simulink model "intgratedMCUSlugs"  (Simulink 7.8)
settings: Solver=FixedStepDiscrete  SolverMode=SingleTasking  StartTime=0.0  StopTime=10.0  FixedStep=0.001  RelTol=1e-3
InitFcn:
  | mcuInit
undefined symbols (not defined in the file): accBiasRateLimit, apSampleTime, barAdjust, baroCutoff, baroCutTemp, baroOffset, baroScale, barTGain1, barTGain2, barTMean1, barTMean2, baseHeight, baseTemp, bda, bde, bdr, bdt, bICda, bICde, bICdr, bICdt, bpan, bPWMpan, bPWMtilt, broll, btilt, changeZoom, controlMCUInit, cubeAccelGain16405, cubeGyroGain16405, cubeMagGain16405, daTrimMax, daTrimMin, deTrimMax, deTrimMin, DiscIntNeverNeededParam, drTrimMax, drTrimMin, dtTrimMax, dtTrimMin, Function_Update, gaind, getCubeData, getGpsMainData, getGPSRawData, getGpsUbloxMainData, getGSLocation, getISRLocation, getMidLevelCommands, getMobileLocation, getPassValues, getRangeOfParams, getRTB, gpsParse, gsRead, gyroBiasRateLimit, hil_getEuler, hil_getRates, hil_getRawRead, hil_getVned ... (+89)
libraries: dsPICdrivers x105, simulink x14, SLUGS_Library x12, aerolibconvert2 x5, aerolibutil x4, aerolibtransform2 x3, dspmtrx3 x3, aerolibobsolete x3
(part 1 of 6)
settings Model: Creator=Marcello G  LastModifiedBy=Marcello G
settings OptimizationCC: OptimizeModelRefInitCode=on  LifeSpan=1
settings DebuggingCC: ParameterPrecisionLossMsg=none
settings HardwareCC: ProdBitPerInt=16  ProdBitPerPointer=16  ProdEndianess=LittleEndian  ProdWordSize=16  ProdHWDeviceType=16-bit Generic
settings RTWCC: SystemTargetFile=dspic.tlc  MakeCommand=make_CreateMPLAB  TemplateMakefile=dspic_pic30_gcc.tmf  PostCodeGenCommand=dsPIC_Compile()  Description=Embedded Target for Microchip dsPIC (real-time)  ProcessScript=dspic_make_rtw_hook
settings CodeAppCC: IgnoreCustomStorageClasses=off
settings STFCustomTargetCC: IncludeMdlTerminateFcn=off  GeneratePreprocessorConditionals=Use local settings  CombineOutputUpdateFcns=on  SuppressErrorStatus=on  ERTCustomFileBanners=on  SupportContinuousTime=off  SupportNonInlinedSFcns=off  SystemTargetFile=dspic.tlc
settings ERTTargetCC: MultiwordLength=2048  ParMdlRefBuildCompliant=off  CompOptLevelCompliant=off  ConcurrentExecutionCompliant=off  IncludeMdlTerminateFcn=off  SuppressErrorStatus=on  ERTFirstTimeCompliant=off  ModelStepFunctionPrototypeControlCompliant=off  CPPClassGenCompliant=off  ExtModeMexFile=ext_serial_win32_comm  InlinedParameterPlacement=NonHierarchical  ERTSrcFileBannerTemplate=dsPIC_code_template.cgt  ERTHdrFileBannerTemplate=dsPIC_code_template.cgt  ERTDataSrcFileTemplate=dsPIC_code_template.cgt  ERTDataHdrFileTemplate=dsPIC_code_template.cgt  ERTCustomFileTemplate=dsPIC_main.tlc  ConvertIfToSwitch=off  SuppressUnreachableDefaultCases=off
settings CustomProperty: DataType=string  Value=D:\MATLAB~1\bin\win64\gmake

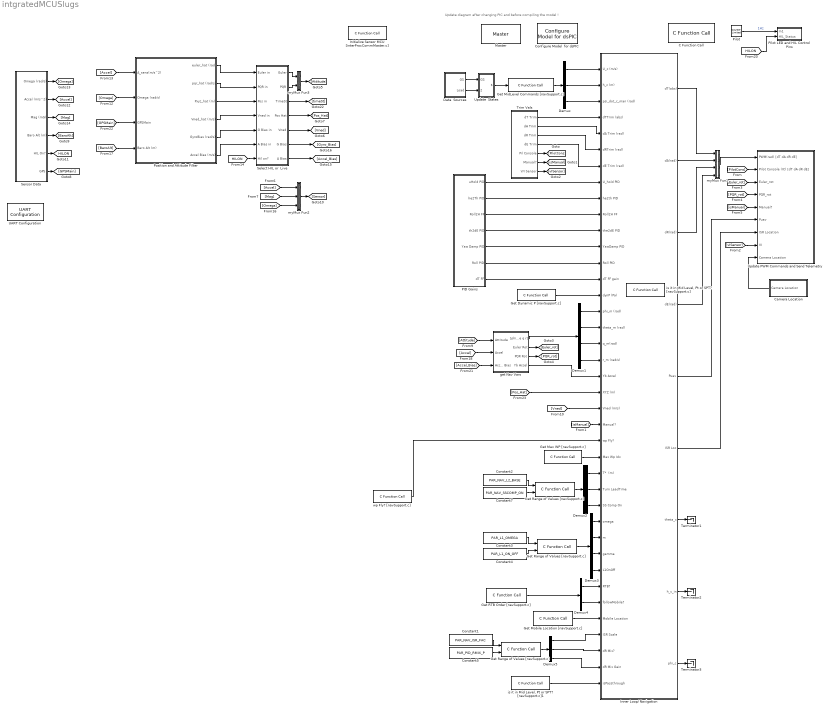
== system intgratedMCUSlugs ==
  note: Update diagram after changing PIC and before compiling the model !
  C Function Call : dsPICdrivers/OTHERS/C Function Call  Tag=dsPIC_dsPIC_CFunctionCall  FctUpdate=None  fctName='Function_Update'  INPUT_SIZE=1  INPUT1=--  INPUT2=--  INPUT3=--  OUTPUT_SIZE=1  OUTPUT1=--  SampleTime=-1  InputType=[]  OutputType=[]  FctDeclaration=extern void Function_Update();  FctCall=Function_Update();  OrderingInOutPopup=None  FctStart=Start Function (Call once and only once)  FctStart_Name='controlMCUInit'  FctStart_Declaration=inline extern void controlMCUInit();  FctStart_Call=controlMCUInit();  FctInit=None  FctInit_Name=Init_Reset  FctInit_Declaration=inline extern void Init_Reset();  FctInit_Call=Init_Reset();  PinDigitalInput=[]  PinDigitalOutput=[]  AnalogueInput=[]
  Camera Location : Subsystem
  Configure Model  for dsPIC : dsPICdrivers/Simulink Configuration/Configure Model  for dsPIC
  Constant1 : Constant  Value=PAR_NAV_ISR_FAC  OutDataTypeStr=uint8
  Constant2 : Constant  Value=PAR_NAV_L2_BASE  OutDataTypeStr=uint8
  Constant3 : Constant  Value=PAR_L1_OMEGA  OutDataTypeStr=uint8
  Constant4 : Constant  Value=PAR_L1_ON_OFF  OutDataTypeStr=uint8
  Constant5 : Constant  Value=PAR_PID_RMIX_P  OutDataTypeStr=uint8
  Constant7 : Constant  Value=PAR_NAV_SSCOMP_ON  OutDataTypeStr=uint8
  Data  Sources : Subsystem
  Demux : Demux  Outputs=3
  Demux1 : Demux
  Demux2 : Demux  Outputs=3
  Demux3 : Demux
  Demux4 : Demux  Outputs=2
  Demux5 : Demux  Outputs=3
  Get Dynamic P [navSupport.c] : dsPICdrivers/OTHERS/C Function Call  Tag=dsPIC_dsPIC_CFunctionCall  FctUpdate=Output Function  fctName='getDynamic'  INPUT_SIZE=1  INPUT1=--  INPUT2=--  INPUT3=--  OUTPUT_SIZE=1  OUTPUT1=real32  SampleTime=.01  InputType=[ ]  OutputType=[ 7 ]  FctDeclaration=extern real32_T getDynamic();  FctCall=%y1 = getDynamic();  OrderingInOutPopup=None  FctStart=None  FctStart_Name=Init_onlyOnce  FctStart_Declaration=inline extern void Init_onlyOnce();  FctStart_Call=Init_onlyOnce();  FctInit=None  FctInit_Name=Init_Reset  FctInit_Declaration=inline extern void Init_Reset();  FctInit_Call=Init_Reset();  PinDigitalInput=[]  PinDigitalOutput=[]  AnalogueInput=[]
  Get Max WP [navSupport.c] : dsPICdrivers/OTHERS/C Function Call  Tag=dsPIC_dsPIC_CFunctionCall  FctUpdate=Output Function  fctName='getMaxWp'  INPUT_SIZE=1  INPUT1=--  INPUT2=--  INPUT3=--  OUTPUT_SIZE=1  OUTPUT1=uint8  SampleTime=.01  InputType=[ ]  OutputType=[ 2 ]  FctDeclaration=extern uint8_T getMaxWp();  FctCall=%y1 = getMaxWp();  OrderingInOutPopup=None  FctStart=None  FctStart_Name=Init_onlyOnce  FctStart_Declaration=inline extern void Init_onlyOnce();  FctStart_Call=Init_onlyOnce();  FctInit=None  FctInit_Name=Init_Reset  FctInit_Declaration=inline extern void Init_Reset();  FctInit_Call=Init_Reset();  PinDigitalInput=[]  PinDigitalOutput=[]  AnalogueInput=[]
  Get MidLevel Commands [navSupport.c] : dsPICdrivers/OTHERS/C Function Call  Tag=dsPIC_dsPIC_CFunctionCall  FctUpdate=Output Function  fctName='getMidLevelCommands'  INPUT_SIZE=1  INPUT1=--  INPUT2=--  INPUT3=--  OUTPUT_SIZE=3  OUTPUT1=real32  SampleTime=.01  InputType=[ ]  OutputType=[ 7 ]  FctDeclaration=extern void getMidLevelCommands(real32_T* y1);  FctCall=getMidLevelCommands(*%y1);  OrderingInOutPopup=Input  FctStart=None  FctStart_Name=Init_onlyOnce  FctStart_Declaration=inline extern void Init_onlyOnce();  FctStart_Call=Init_onlyOnce();  FctInit=None  FctInit_Name=Init_Reset  FctInit_Declaration=inline extern void Init_Reset();  FctInit_Call=Init_Reset();  PinDigitalInput=[]  PinDigitalOutput=[]  AnalogueInput=[]
  "Get Mobile Location [navSupport.c] " : dsPICdrivers/OTHERS/C Function Call  Tag=dsPIC_dsPIC_CFunctionCall  FctUpdate=Output Function  fctName='getMobileLocation'  INPUT_SIZE=1  INPUT1=--  INPUT2=--  INPUT3=--  OUTPUT_SIZE=2  OUTPUT1=real32  SampleTime=.01  InputType=[ ]  OutputType=[ 7 ]  FctDeclaration=extern void getMobileLocation(real32_T* y1);  FctCall=getMobileLocation(*%y1);  OrderingInOutPopup=None  FctStart=None  FctStart_Name=Init_onlyOnce  FctStart_Declaration=inline extern void Init_onlyOnce();  FctStart_Call=Init_onlyOnce();  FctInit=None  FctInit_Name=Init_Reset  FctInit_Declaration=inline extern void Init_Reset();  FctInit_Call=Init_Reset();  PinDigitalInput=[]  PinDigitalOutput=[]  AnalogueInput=[]
  Get RTB Order [navSupport.c] : dsPICdrivers/OTHERS/C Function Call  Tag=dsPIC_dsPIC_CFunctionCall  FctUpdate=Output Function  fctName='getRTB'  INPUT_SIZE=1  INPUT1=--  INPUT2=--  INPUT3=--  OUTPUT_SIZE=2  OUTPUT1=uint8  SampleTime=.01  InputType=[ ]  OutputType=[ 2 ]  FctDeclaration=extern void getRTB(uint8_T* y1);  FctCall=getRTB(*%y1);  OrderingInOutPopup=None  FctStart=None  FctStart_Name=Init_onlyOnce  FctStart_Declaration=inline extern void Init_onlyOnce();  FctStart_Call=Init_onlyOnce();  FctInit=None  FctInit_Name=Init_Reset  FctInit_Declaration=inline extern void Init_Reset();  FctInit_Call=Init_Reset();  PinDigitalInput=[]  PinDigitalOutput=[]  AnalogueInput=[]
  Get Range of Values [navSupport.c] : dsPICdrivers/OTHERS/C Function Call  Tag=dsPIC_dsPIC_CFunctionCall  FctUpdate=Output Function  fctName='getRangeOfParams'  INPUT_SIZE=1  INPUT1=uint8  INPUT2=uint8  INPUT3=--  OUTPUT_SIZE=3  OUTPUT1=real32  SampleTime=.01  InputType=[ 2 2 ]  OutputType=[ 7 ]  FctDeclaration=extern void getRangeOfParams(uint8_T u1, uint8_T u2,real32_T* y1);  FctCall=getRangeOfParams(%u1, %u2, *%y1);  OrderingInOutPopup=None  FctStart=None  FctStart_Name=Init_onlyOnce  FctStart_Declaration=inline extern void Init_onlyOnce();  FctStart_Call=Init_onlyOnce();  FctInit=None  FctInit_Name=Init_Reset  FctInit_Declaration=inline extern void Init_Reset();  FctInit_Call=Init_Reset();  PinDigitalInput=[]  PinDigitalOutput=[]  AnalogueInput=[]
  "Get Range of Values [navSupport.c] " : dsPICdrivers/OTHERS/C Function Call  Tag=dsPIC_dsPIC_CFunctionCall  FctUpdate=Output Function  fctName='getRangeOfParams'  INPUT_SIZE=1  INPUT1=uint8  INPUT2=uint8  INPUT3=--  OUTPUT_SIZE=4  OUTPUT1=real32  SampleTime=.01  InputType=[ 2 2 ]  OutputType=[ 7 ]  FctDeclaration=extern void getRangeOfParams(uint8_T u1, uint8_T u2,real32_T* y1);  FctCall=getRangeOfParams(%u1, %u2, *%y1);  OrderingInOutPopup=None  FctStart=None  FctStart_Name=Init_onlyOnce  FctStart_Declaration=inline extern void Init_onlyOnce();  FctStart_Call=Init_onlyOnce();  FctInit=None  FctInit_Name=Init_Reset  FctInit_Declaration=inline extern void Init_Reset();  FctInit_Call=Init_Reset();  PinDigitalInput=[]  PinDigitalOutput=[]  AnalogueInput=[]
  "Get Range of Values [navSupport.c]   " : dsPICdrivers/OTHERS/C Function Call  Tag=dsPIC_dsPIC_CFunctionCall  FctUpdate=Output Function  fctName='getRangeOfParams'  INPUT_SIZE=1  INPUT1=uint8  INPUT2=uint8  INPUT3=--  OUTPUT_SIZE=3  OUTPUT1=real32  SampleTime=.01  InputType=[ 2 2 ]  OutputType=[ 7 ]  FctDeclaration=extern void getRangeOfParams(uint8_T u1, uint8_T u2,real32_T* y1);  FctCall=getRangeOfParams(%u1, %u2, *%y1);  OrderingInOutPopup=None  FctStart=None  FctStart_Name=Init_onlyOnce  FctStart_Declaration=inline extern void Init_onlyOnce();  FctStart_Call=Init_onlyOnce();  FctInit=None  FctInit_Name=Init_Reset  FctInit_Declaration=inline extern void Init_Reset();  FctInit_Call=Init_Reset();  PinDigitalInput=[]  PinDigitalOutput=[]  AnalogueInput=[]
  Initialize Sensor MCU [interProcCommMaster.c] : dsPICdrivers/OTHERS/C Function Call  Tag=dsPIC_dsPIC_CFunctionCall  FctUpdate=None  fctName='Function_Update'  INPUT_SIZE=1  INPUT1=--  INPUT2=--  INPUT3=--  OUTPUT_SIZE=1  OUTPUT1=--  SampleTime=inf  InputType=[]  OutputType=[]  FctDeclaration=extern void Function_Update();  FctCall=Function_Update();  OrderingInOutPopup=None  FctStart=Start Function (Call once and only once)  FctStart_Name='sensorMCUInit'  FctStart_Declaration=inline extern void sensorMCUInit();  FctStart_Call=sensorMCUInit();  FctInit=None  FctInit_Name=Init_Reset  FctInit_Declaration=inline extern void Init_Reset();  FctInit_Call=Init_Reset();  PinDigitalInput=[]  PinDigitalOutput=[]  AnalogueInput=[]
  Inner Loop/ Navigation : Subsystem
  Master : dsPICdrivers/Master  Tag=dsPIC_MASTER  Priority=1  TimeStepType=Timer1  picType=33fJ256MC710  fcy=40000000  Quartz_33f=12e6  PLLActive_33f=on  fcyDesired_33f=40000000  tmr1="[1  39999  0]"  tmr1Info="Time Step : 0.001  ;   Error : 0%  PR1=39999"  tmr2345="[8  0  0  0  0  0  0  0]"  tmr2345cfg=[-1 -1 -1 -1 -1 -1 -1 -1]  IOautoConf=on  typePort="[ 0   0   0   0   0   0   0   0   0   0   0   0   0   0   9   0   0   0   0   0   0   0  10   0   8   8   8   8   0   0   0   0   0   0   0   0   0   0   0   0   0   0   0   0   0   0   0   0   0   0   9   0   0   0   0   0   6   6   6   6   6   0   6   6  11   0  11   0  11   0  11   0   0  10   0   0   0   0   0   0   0   0   4   0   0   0   0   0   0   0   0   0   0   0   0   0   0   0   0   0   0   0   0  10  10  10   0   0   0   0   0  10 ]"  TRIS="[ 65535  65471  65535  65535  65023  65535  31871 ]"  ADPCFG=2097216  MasterBusyPort=None  MasterOverloadPort=None  FOSC=External Clock  ClockSwitchMonitor=Both disabled  TempProtection_33f=TEMP_ON  FPBOR=<empty>  PWRT=disable  MCLR=<empty>  ICD=ICS_PGD2  JTAGEN=JTAGEN_OFF  PowerSave=off  OverrideFcy=off  NewFcy=1e6  PR2345="[65535  65535  65535  65535  65535  65535  65535  65535]"
  PID Gains : Subsystem
  Pilot : simulink/Sources/Counter Limited  uplimit=1  tsamp=1.0
  Pilot LED and HIL Control Pins : Subsystem
  Position and Attitude Filter : Subsystem
  Select HIL or  Live : Subsystem
  Sensor Data : Subsystem
  Terminator1 : Terminator
  Terminator2 : Terminator
  Terminator3 : Terminator
  Trim Vals : Subsystem
  UART Configuration : dsPICdrivers/Serial PORT/UART Configuration  Tag=dsPIC_config_UART  Priority=2  UART=1  proposed_BAUD=38400  BAUD=38400  ALT_TX_RX=on  InterruptTxWhen=When Transmit Buffer is empty  TXInterruptPri=1  TxBufferSize=32  TXEN=off  InterruptRxWhen=When a character is received  RXInterruptPri=2  RxBufferSize=32  DoNotImplementRxInterrupt=on  DoNotImplementTxInterrupt=on  UxBRG=64  Info="UxBRG = 64   ||  Real Baud : 38462   ||  % error : 0.16026  ||  max 3.8462 Bytes / Step"  RealBaud=0  ERROR=0.16026  BYTES_STEP=3.8462
  Update  States : Subsystem
  Update PWM Commands and Send Telemetry : Subsystem
  get Nav Vars : Subsystem
  "is it in Mid Level, Pt or SPT? [navSupport.c]" : dsPICdrivers/OTHERS/C Function Call  Tag=dsPIC_dsPIC_CFunctionCall  FctUpdate=Output Function  fctName='isPassthrough'  INPUT_SIZE=1  INPUT1=--  INPUT2=--  INPUT3=--  OUTPUT_SIZE=1  OUTPUT1=uint8  SampleTime=0.01  InputType=[ ]  OutputType=[ 2 ]  FctDeclaration=extern uint8_T isPassthrough();  FctCall=%y1 = isPassthrough();  OrderingInOutPopup=None  FctStart=None  FctStart_Name=Init_onlyOnce  FctStart_Declaration=inline extern void Init_onlyOnce();  FctStart_Call=Init_onlyOnce();  FctInit=None  FctInit_Name=Init_Reset  FctInit_Declaration=inline extern void Init_Reset();  FctInit_Call=Init_Reset();  PinDigitalInput=[]  PinDigitalOutput=[]  AnalogueInput=[]
  "is it in Mid Level, Pt or SPT? [navSupport.c]1" : dsPICdrivers/OTHERS/C Function Call  Tag=dsPIC_dsPIC_CFunctionCall  FctUpdate=Output Function  fctName='isPassthrough'  INPUT_SIZE=1  INPUT1=--  INPUT2=--  INPUT3=--  OUTPUT_SIZE=1  OUTPUT1=uint8  SampleTime=0.01  InputType=[ ]  OutputType=[ 2 ]  FctDeclaration=extern uint8_T isPassthrough();  FctCall=%y1 = isPassthrough();  OrderingInOutPopup=None  FctStart=None  FctStart_Name=Init_onlyOnce  FctStart_Declaration=inline extern void Init_onlyOnce();  FctStart_Call=Init_onlyOnce();  FctInit=None  FctInit_Name=Init_Reset  FctInit_Declaration=inline extern void Init_Reset();  FctInit_Call=Init_Reset();  PinDigitalInput=[]  PinDigitalOutput=[]  AnalogueInput=[]
  myMux Fun1 : MATLAB Function  TreatAsAtomicUnit=on
  myMux Fun2 : MATLAB Function  TreatAsAtomicUnit=on
  myMux Fun3 : MATLAB Function  TreatAsAtomicUnit=on
  wp Fly? [navSupport.c] : dsPICdrivers/OTHERS/C Function Call  Tag=dsPIC_dsPIC_CFunctionCall  FctUpdate=Output Function  fctName='isWpFly'  INPUT_SIZE=1  INPUT1=--  INPUT2=--  INPUT3=--  OUTPUT_SIZE=1  OUTPUT1=uint8  SampleTime=.01  InputType=[ ]  OutputType=[ 2 ]  FctDeclaration=extern uint8_T isWpFly();  FctCall=%y1 = isWpFly();  OrderingInOutPopup=None  FctStart=None  FctStart_Name=Init_onlyOnce  FctStart_Declaration=inline extern void Init_onlyOnce();  FctStart_Call=Init_onlyOnce();  FctInit=None  FctInit_Name=Init_Reset  FctInit_Declaration=inline extern void Init_Reset();  FctInit_Call=Init_Reset();  PinDigitalInput=[]  PinDigitalOutput=[]  AnalogueInput=[]
  tag scope: HILON=global
  wires:
  Pilot/1 -> Pilot LED and HIL Control Pins/1(In1)  "1Hz"
  Data  Sources/1(GS) -> Update  States/1(GS)
  Data  Sources/2(Load) -> Update  States/2(Load)
  Demux/1 -> Inner Loop/ Navigation/1(U_c (m/s))
  Demux/2 -> Inner Loop/ Navigation/2(h_c (m))
  Demux/3 -> Inner Loop/ Navigation/3(psi_dot_c_man (rad))
  Get MidLevel Commands [navSupport.c]/1 -> Demux/1
  Trim Vals/4(dE Trim) -> Inner Loop/ Navigation/7(dE Trim (rad))
  Trim Vals/1(dT Trim) -> Inner Loop/ Navigation/4(dTTrim (abs))
  Trim Vals/2(dA Trim) -> Inner Loop/ Navigation/5(dA Trim (rad))
  Trim Vals/3(dR Trim) -> Inner Loop/ Navigation/6(dRTrim (rad))
  PID Gains/1(uHold PID) -> Inner Loop/ Navigation/8(U_hold PID)
  PID Gains/2(he2Th PID) -> Inner Loop/ Navigation/9(he2th PID)
  PID Gains/4(th2dE PID) -> Inner Loop/ Navigation/11(the2dE PID)
  PID Gains/5(Yaw Damp PID) -> Inner Loop/ Navigation/12(YawDamp PID)
  PID Gains/6(Roll PID) -> Inner Loop/ Navigation/13("Roll PID ")
  Get Dynamic P [navSupport.c]/1 -> Inner Loop/ Navigation/15(dynP (Pa))
  get Nav Vars/1("[phi the q r]") -> Demux1/1
  Demux1/1 -> Inner Loop/ Navigation/16(phi_m (rad))
  Demux1/2 -> Inner Loop/ Navigation/17(theta_m (rad))
  Get Max WP [navSupport.c]/1 -> Inner Loop/ Navigation/25(Max Wp Idx)
  Update  States/1($) -> Get MidLevel Commands [navSupport.c]/1
  wp Fly? [navSupport.c]/1 -> Inner Loop/ Navigation/24(wp Fly?)
  Inner Loop/ Navigation/7(theta_c) -> Terminator1/1
  Inner Loop/ Navigation/8(h_c_in) -> Terminator2/1
  Inner Loop/ Navigation/9(phi_c) -> Terminator3/1
  Demux1/4 -> Inner Loop/ Navigation/19(r_m (rad/s))
  Demux1/3 -> Inner Loop/ Navigation/18(q_m(rad))
  Trim Vals/5(Pil Console) -> [PilotCons]
  Inner Loop/ Navigation/1(dT(abs)) -> myMux Fun1/1(u1)
  Inner Loop/ Navigation/2(dA(rad)) -> myMux Fun1/2(u2)
  Inner Loop/ Navigation/3(dR(rad)) -> myMux Fun1/3(u3)
  Inner Loop/ Navigation/4(dE(rad)) -> myMux Fun1/4(u4)
  [PilotCons] -> Update PWM Commands and Send Telemetry/2(Pilot Console (IC) [dT dA dR dE])
  myMux Fun1/1(y) -> Update PWM Commands and Send Telemetry/1(PWM(rad) [dT dA dR dE])
  get Nav Vars/2(Euler Rot) -> [Euler_rot]
  get Nav Vars/3(PQR Rot) -> [PQR_rot]
  [Euler_rot] -> Update PWM Commands and Send Telemetry/3(Euler_rot)
  [PQR_rot] -> Update PWM Commands and Send Telemetry/4(PQR_rot)
  get Nav Vars/4(Yb Accel) -> Inner Loop/ Navigation/20(Yb Accel)
  [Pos_Hat] -> Inner Loop/ Navigation/21(XYZ (m))
  [Vned] -> Inner Loop/ Navigation/22(Vned (m/s))
  PID Gains/3(Roll2H FF) -> Inner Loop/ Navigation/10(Roll2H FF)
  Demux2/1 -> Inner Loop/ Navigation/26(T*  (m))
  Demux2/2 -> Inner Loop/ Navigation/27(Turn LeadTime)
  Demux2/3 -> Inner Loop/ Navigation/28(SS Comp On)
  Constant2/1 -> Get Range of Values [navSupport.c]/1
  Constant7/1 -> Get Range of Values [navSupport.c]/2
  Get Range of Values [navSupport.c]/1 -> Demux2/1
  PID Gains/7(dT FF) -> Inner Loop/ Navigation/14(dT FF gain)
  Constant3/1 -> "Get Range of Values [navSupport.c] "/1
  Constant4/1 -> "Get Range of Values [navSupport.c] "/2
  "Get Range of Values [navSupport.c] "/1 -> Demux3/1
  Demux3/1 -> Inner Loop/ Navigation/29(omega)
  Demux3/2 -> Inner Loop/ Navigation/30(m)
  Demux3/3 -> Inner Loop/ Navigation/31(gamma)
  Demux3/4 -> Inner Loop/ Navigation/32(L1OnOff)
  Trim Vals/6(Manual?) -> [isManual]
  [isManual] -> Inner Loop/ Navigation/23(Manual?)
  [isManual] -> Update PWM Commands and Send Telemetry/5(Manual?)
  Get RTB Order [navSupport.c]/1 -> Demux4/1
  Demux4/1 -> Inner Loop/ Navigation/33(RTB?)
  Demux4/2 -> Inner Loop/ Navigation/34(followMobile?)
  "Get Mobile Location [navSupport.c] "/1 -> Inner Loop/ Navigation/35(Mobile Location)
  Inner Loop/ Navigation/5("Puav ") -> Update PWM Commands and Send Telemetry/6(Puav)
  Inner Loop/ Navigation/6(ISR Loc) -> Update PWM Commands and Send Telemetry/7(ISR Location)
  Trim Vals/7(V/I Sensor) -> [vISensor]
  [vISensor] -> Update PWM Commands and Send Telemetry/8(VI)
  Constant1/1 -> "Get Range of Values [navSupport.c]   "/1
  Constant5/1 -> "Get Range of Values [navSupport.c]   "/2
  "Get Range of Values [navSupport.c]   "/1 -> Demux5/1
  Demux5/1 -> Inner Loop/ Navigation/36(ISR Scale)
  Demux5/2 -> Inner Loop/ Navigation/37(dR Mix?)
  Demux5/3 -> Inner Loop/ Navigation/38(dR Mix Gain)
  Camera Location/1(Camera Location) -> Update PWM Commands and Send Telemetry/9(Camera Location)
  "is it in Mid Level, Pt or SPT? [navSupport.c]1"/1 -> Inner Loop/ Navigation/39(isPassthrough)
  myMux Fun3/1(y) -> [Attitude]
  Select HIL or  Live/1(Euler) -> myMux Fun3/1(u1)
  Select HIL or  Live/2(PQR) -> myMux Fun3/2(u2)
  Select HIL or  Live/3(TimeSt) -> [timeSt]
  Sensor Data/2(Accel (m/s^2)) -> [Accel]
  Sensor Data/1(Omega (rad/s)) -> [Omega]
  Sensor Data/3(Mag (mG)) -> [Mag]
  Sensor Data/4(Baro Alt (m)) -> [BaroAlt]
  Sensor Data/5(HIL On?) -> [HILON]
  Sensor Data/6(GPS) -> [GPSMain]
  [HILON] -> Select HIL or  Live/7(Hil on?)
  [Omega] -> Position and Attitude Filter/2(Omega (rad/s))
  [Accel] -> Position and Attitude Filter/1(A_sens(m/s^2))
  Position and Attitude Filter/1(euler_hat (rad)) -> Select HIL or  Live/1(Euler in)
  Position and Attitude Filter/2(pqr_hat (rad/s)) -> Select HIL or  Live/2(PQR in)
  Position and Attitude Filter/3(Pxyz_hat (m)) -> Select HIL or  Live/3(Pos in)
  Position and Attitude Filter/4(Vned_hat (m/s)) -> Select HIL or  Live/4(Vned in)
  Position and Attitude Filter/5(GyroBias (rad/s)) -> Select HIL or  Live/5(G Bias in)
  Position and Attitude Filter/6(Accel Bias (m/s)) -> Select HIL or  Live/6(A Bias in)
  [GPSMain] -> Position and Attitude Filter/3(GPSMain)
  [BaroAlt] -> Position and Attitude Filter/4(Baro Alt (m))
  myMux Fun2/1(y) -> [Sensor]
  [Accel] -> myMux Fun2/1(u1)
  [Mag] -> myMux Fun2/2(u2)
  [Omega] -> myMux Fun2/3(u3)
  [Accel] -> get Nav Vars/2(Accel)
  [Attitude] -> get Nav Vars/1(Attitude)
  Select HIL or  Live/7(A Bias) -> [Accel_Bias]
  [Accel_Bias] -> get Nav Vars/3(Accel. Bias)
  Select HIL or  Live/5(Vned) -> [Vned]
  Select HIL or  Live/4(Pos Hat) -> [Pos_Hat]
  [HILON] -> Pilot LED and HIL Control Pins/2(HIL_Status)
  Select HIL or  Live/6(G Bias) -> [Gyro_Bias]

== system intgratedMCUSlugs/Camera Location ==
  Constant : Constant  Value=0  OutDataTypeStr=single
  Constant6 : Constant  Value=PAR_CAM_X  OutDataTypeStr=uint8
  Constant8 : Constant  Value=PAR_CAM_Z  OutDataTypeStr=uint8
  Demux6 : Demux  Outputs=2
  "Get Range of Values [navSupport.c]     " : dsPICdrivers/OTHERS/C Function Call  Tag=dsPIC_dsPIC_CFunctionCall  FctUpdate=Output Function  fctName='getRangeOfParams'  INPUT_SIZE=1  INPUT1=uint8  INPUT2=uint8  INPUT3=--  OUTPUT_SIZE=2  OUTPUT1=real32  SampleTime=.01  InputType=[ 2 2 ]  OutputType=[ 7 ]  FctDeclaration=extern void getRangeOfParams(uint8_T u1, uint8_T u2,real32_T* y1);  FctCall=getRangeOfParams(%u1, %u2, *%y1);  OrderingInOutPopup=None  FctStart=None  FctStart_Name=Init_onlyOnce  FctStart_Declaration=inline extern void Init_onlyOnce();  FctStart_Call=Init_onlyOnce();  FctInit=None  FctInit_Name=Init_Reset  FctInit_Declaration=inline extern void Init_Reset();  FctInit_Call=Init_Reset();  PinDigitalInput=[]  PinDigitalOutput=[]  AnalogueInput=[]
  myMux Fun4 : MATLAB Function  TreatAsAtomicUnit=on
  Camera Location : Outport
  wires:
  Constant6/1 -> "Get Range of Values [navSupport.c]     "/1
  Constant8/1 -> "Get Range of Values [navSupport.c]     "/2
  "Get Range of Values [navSupport.c]     "/1 -> Demux6/1
  Demux6/1 -> myMux Fun4/1(u1)
  Demux6/2 -> myMux Fun4/3(u3)
  Constant/1 -> myMux Fun4/2(u2)
  myMux Fun4/1(y) -> Camera Location/1

== system intgratedMCUSlugs/Data  Sources ==
  Compute Load : Subsystem
  Data from GS [mavlinkCommsControlMcu.c] : dsPICdrivers/OTHERS/C Function Call  Tag=dsPIC_dsPIC_CFunctionCall  FctUpdate=Output Function  fctName='gsRead'  INPUT_SIZE=1  INPUT1=--  INPUT2=--  INPUT3=--  OUTPUT_SIZE=202  OUTPUT1=uint8  SampleTime=.01  InputType=[ ]  OutputType=[ 2 ]  FctDeclaration=extern void gsRead(uint8_T* y1);  FctCall=gsRead(*%y1);  OrderingInOutPopup=None  FctStart=None  FctStart_Name=Init_onlyOnce  FctStart_Declaration=inline extern void Init_onlyOnce();  FctStart_Call=Init_onlyOnce();  FctInit=None  FctInit_Name=Init_Reset  FctInit_Declaration=inline extern void Init_Reset();  FctInit_Call=Init_Reset();  PinDigitalInput=[]  PinDigitalOutput=[]  AnalogueInput=[]
  GS : Outport
  Load : Outport  Port=2
  wires:
  Data from GS [mavlinkCommsControlMcu.c]/1 -> GS/1
  Compute Load/1(Load (%)) -> Load/1

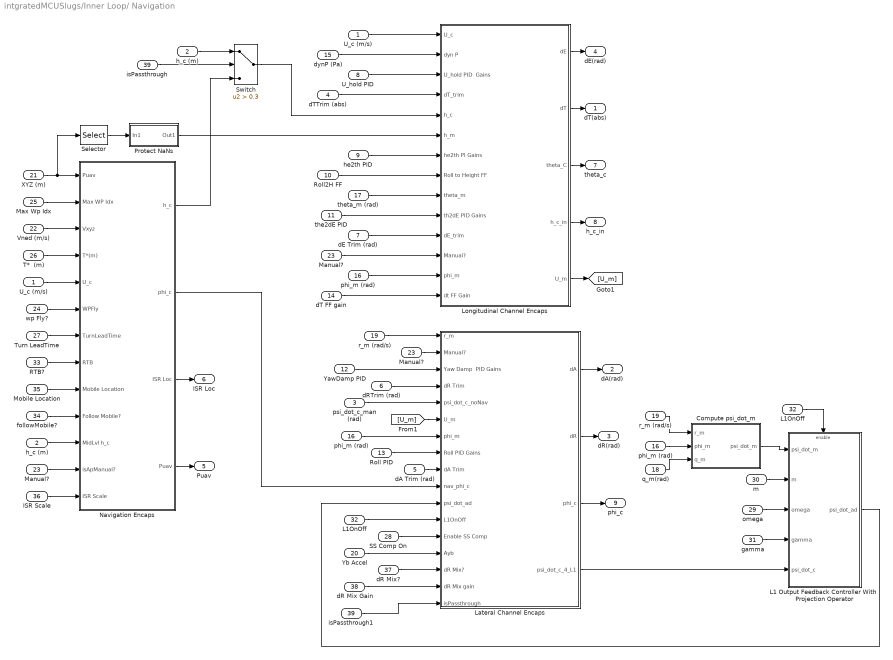
== system intgratedMCUSlugs/Inner Loop/ Navigation ==
  U_c (m/s) : Inport
  h_c (m) : Inport  Port=2
  psi_dot_c_man (rad) : Inport  Port=3
  dTTrim (abs) : Inport  Port=4
  dA Trim (rad) : Inport  Port=5
  dRTrim (rad) : Inport  Port=6
  dE Trim (rad) : Inport  Port=7
  U_hold PID : Inport  Port=8
  he2th PID : Inport  Port=9
  Roll2H FF : Inport  Port=10
  the2dE PID : Inport  Port=11
  YawDamp PID : Inport  Port=12
  "Roll PID " : Inport  Port=13
  dT FF gain : Inport  Port=14
  dynP (Pa) : Inport  Port=15
  phi_m (rad) : Inport  Port=16
  theta_m (rad) : Inport  Port=17
  q_m(rad) : Inport  Port=18
  r_m (rad/s) : Inport  Port=19
  Yb Accel : Inport  Port=20
  XYZ (m) : Inport  Port=21
  Vned (m/s) : Inport  Port=22
  Manual? : Inport  Port=23
  wp Fly? : Inport  Port=24
  Max Wp Idx : Inport  Port=25
  T*  (m) : Inport  Port=26
  Turn LeadTime : Inport  Port=27
  SS Comp On : Inport  Port=28
  omega : Inport  Port=29
  m : Inport  Port=30
  gamma : Inport  Port=31
  L1OnOff : Inport  Port=32
  RTB? : Inport  Port=33
  followMobile? : Inport  Port=34
  Mobile Location : Inport  Port=35
  ISR Scale : Inport  Port=36
  dR Mix? : Inport  Port=37
  dR Mix Gain : Inport  Port=38
  isPassthrough : Inport  Port=39
  Compute psi_dot_m : Subsystem
  L1 Output Feedback Controller With  Projection Operator : Subsystem  TreatAsAtomicUnit=on
  "L1OnOff " : InportShadow  Port=32
  Lateral Channel Encaps : Subsystem  TreatAsAtomicUnit=on
  Longitudinal Channel Encaps : Subsystem  TreatAsAtomicUnit=on
  "Manual? " : InportShadow  Port=23
  "Manual?  " : InportShadow  Port=23
  Navigation Encaps : Subsystem  TreatAsAtomicUnit=on
  Protect NaNs : Subsystem
  Selector : Selector  InputPortWidth=3  IndexOptions=Index vector (dialog)  Indices=[3]  OutputSizes=1
  Switch : Switch  Criteria=u2 > Threshold  Threshold=0.3  OutDataTypeStr=Inherit: Inherit via back propagation  InputSameDT=on
  "U_c (m/s) " : InportShadow  Port=1
  "h_c (m) " : InportShadow  Port=2
  isPassthrough1 : InportShadow  Port=39
  "phi_m (rad) " : InportShadow  Port=16
  "phi_m (rad)   " : InportShadow  Port=16
  "r_m (rad/s) " : InportShadow  Port=19
  dT(abs) : Outport
  dA(rad) : Outport  Port=2
  dR(rad) : Outport  Port=3
  dE(rad) : Outport  Port=4
  "Puav " : Outport  Port=5
  ISR Loc : Outport  Port=6
  theta_c : Outport  Port=7
  h_c_in : Outport  Port=8
  phi_c : Outport  Port=9
  wires:
  Manual?/1 -> Longitudinal Channel Encaps/12(Manual?)
  U_c (m/s)/1 -> Longitudinal Channel Encaps/1(U_c)
  dynP (Pa)/1 -> Longitudinal Channel Encaps/2(dyn P)
  Longitudinal Channel Encaps/1(dE) -> dE(rad)/1
  U_hold PID/1 -> Longitudinal Channel Encaps/3(U_hold PID  Gains)
  dTTrim (abs)/1 -> Longitudinal Channel Encaps/4(dT_trim)
  Longitudinal Channel Encaps/2(dT) -> dT(abs)/1
  Selector/1 -> Protect NaNs/1(In1)
  he2th PID/1 -> Longitudinal Channel Encaps/7(he2th PI Gains)
  theta_m (rad)/1 -> Longitudinal Channel Encaps/9(theta_m)
  Longitudinal Channel Encaps/3(theta_C) -> theta_c/1
  the2dE PID/1 -> Longitudinal Channel Encaps/10(th2dE PID Gains)
  dE Trim (rad)/1 -> Longitudinal Channel Encaps/11(dE_trim)
  Longitudinal Channel Encaps/4(h_c_in) -> h_c_in/1
  r_m (rad/s)/1 -> Lateral Channel Encaps/1(r_m)
  YawDamp PID/1 -> Lateral Channel Encaps/3(Yaw Damp  PID Gains)
  dRTrim (rad)/1 -> Lateral Channel Encaps/4(dR Trim)
  Lateral Channel Encaps/2(dR) -> dR(rad)/1
  psi_dot_c_man (rad)/1 -> Lateral Channel Encaps/5(psi_dot_c_noNav)
  phi_m (rad)/1 -> Lateral Channel Encaps/7(phi_m)
  Lateral Channel Encaps/3(phi_c) -> phi_c/1
  "Roll PID "/1 -> Lateral Channel Encaps/8(Roll PID Gains)
  dA Trim (rad)/1 -> Lateral Channel Encaps/9(dA Trim)
  Longitudinal Channel Encaps/5(U_m) -> [U_m]
  XYZ (m)/1 -> Selector/1, Navigation Encaps/1(Puav)
  Max Wp Idx/1 -> Navigation Encaps/2(Max WP Idx)
  Vned (m/s)/1 -> Navigation Encaps/3(Vxyz)
  Compute psi_dot_m/1(psi_dot_m) -> L1 Output Feedback Controller With  Projection Operator/1(psi_dot_m)
  m/1 -> L1 Output Feedback Controller With  Projection Operator/2(m)
  omega/1 -> L1 Output Feedback Controller With  Projection Operator/3(omega)
  gamma/1 -> L1 Output Feedback Controller With  Projection Operator/4(gamma)
  "r_m (rad/s) "/1 -> Compute psi_dot_m/1(r_m)
  "phi_m (rad) "/1 -> Compute psi_dot_m/2(phi_m)
  q_m(rad)/1 -> Compute psi_dot_m/3(q_m)
  L1OnOff/1 -> L1 Output Feedback Controller With  Projection Operator/Enable
  L1 Output Feedback Controller With  Projection Operator/1(psi_dot_ad) -> Lateral Channel Encaps/11(psi_dot_ad)
  "L1OnOff "/1 -> Lateral Channel Encaps/12(L1OnOff)
  "phi_m (rad)   "/1 -> Longitudinal Channel Encaps/13(phi_m)
  dT FF gain/1 -> Longitudinal Channel Encaps/14(dt FF Gain)
  Lateral Channel Encaps/1(dA) -> dA(rad)/1
  SS Comp On/1 -> Lateral Channel Encaps/13(Enable SS Comp)
  Yb Accel/1 -> Lateral Channel Encaps/14(Ayb)
  Lateral Channel Encaps/4(psi_dot_c_4_L1) -> L1 Output Feedback Controller With  Projection Operator/5(psi_dot_c)
  Protect NaNs/1(Out1) -> Longitudinal Channel Encaps/6(h_m)
  [U_m] -> Lateral Channel Encaps/6(U_m)
  "Manual?  "/1 -> Lateral Channel Encaps/2(Manual?)
  Roll2H FF/1 -> Longitudinal Channel Encaps/8(Roll to Height FF)
  Navigation Encaps/2(phi_c) -> Lateral Channel Encaps/10(nav_phi_c)
  T*  (m)/1 -> Navigation Encaps/4(T*(m))
  "U_c (m/s) "/1 -> Navigation Encaps/5(U_c)
  wp Fly?/1 -> Navigation Encaps/6(WPFly)
  Turn LeadTime/1 -> Navigation Encaps/7(TurnLeadTime)
  RTB?/1 -> Navigation Encaps/8(RTB)
  Mobile Location/1 -> Navigation Encaps/9(Mobile Location)
  followMobile?/1 -> Navigation Encaps/10(Follow Mobile?)
  "h_c (m) "/1 -> Navigation Encaps/11(MidLvl h_c)
  "Manual? "/1 -> Navigation Encaps/12(isApManual?)
  Navigation Encaps/3(ISR Loc) -> ISR Loc/1
  Navigation Encaps/4("Puav ") -> "Puav "/1
  dR Mix Gain/1 -> Lateral Channel Encaps/16(dR Mix gain)
  dR Mix?/1 -> Lateral Channel Encaps/15(dR Mix?)
  ISR Scale/1 -> Navigation Encaps/13(ISR Scale)
  isPassthrough/1 -> Switch/2
  h_c (m)/1 -> Switch/1
  Switch/1 -> Longitudinal Channel Encaps/5(h_c)
  Navigation Encaps/1(h_c) -> Switch/3
  isPassthrough1/1 -> Lateral Channel Encaps/17(isPassthrough)

== system intgratedMCUSlugs/PID Gains ==
  Constant1 : Constant  Value=PAR_PID_AIRSPEED_P  OutDataTypeStr=uint8
  Constant10 : Constant  Value=PAR_PID_PITCH_FO_P  OutDataTypeStr=uint8
  Constant11 : Constant  Value=PAR_PID_PITCH_FO_I  OutDataTypeStr=uint8
  Constant12 : Constant  Value=PAR_PID_PITC_DT_FF  OutDataTypeStr=uint8
  Constant2 : Constant  Value=PAR_PID_ROLL_CON_P  OutDataTypeStr=uint8
  Constant3 : Constant  Value=PAR_PID_ROLL_CON_D  OutDataTypeStr=uint8
  Constant4 : Constant  Value=PAR_PID_YAW_DAMP_P  OutDataTypeStr=uint8
  Constant5 : Constant  Value=PAR_PID_YAW_DAMP_D  OutDataTypeStr=uint8
  Constant6 : Constant  Value=PAR_PID_HE_TO_PI_P  OutDataTypeStr=uint8
  Constant7 : Constant  Value=PAR_PID_AIRSPEED_D  OutDataTypeStr=uint8
  Constant8 : Constant  Value=PAR_PID_HE_TO_PI_I  OutDataTypeStr=uint8
  Constant9 : Constant  Value=PAR_PID_HEI_ERR_FF  OutDataTypeStr=uint8
  Get Range of Values [navSupport.c] : dsPICdrivers/OTHERS/C Function Call  Tag=dsPIC_dsPIC_CFunctionCall  FctUpdate=Output Function  fctName='getRangeOfParams'  INPUT_SIZE=1  INPUT1=uint8  INPUT2=uint8  INPUT3=--  OUTPUT_SIZE=3  OUTPUT1=real32  SampleTime=.01  InputType=[ 2 2 ]  OutputType=[ 7 ]  FctDeclaration=extern void getRangeOfParams(uint8_T u1, uint8_T u2,real32_T* y1);  FctCall=getRangeOfParams(%u1, %u2, *%y1);  OrderingInOutPopup=None  FctStart=None  FctStart_Name=Init_onlyOnce  FctStart_Declaration=inline extern void Init_onlyOnce();  FctStart_Call=Init_onlyOnce();  FctInit=None  FctInit_Name=Init_Reset  FctInit_Declaration=inline extern void Init_Reset();  FctInit_Call=Init_Reset();  PinDigitalInput=[]  PinDigitalOutput=[]  AnalogueInput=[]
  "Get Range of Values [navSupport.c] " : dsPICdrivers/OTHERS/C Function Call  Tag=dsPIC_dsPIC_CFunctionCall  FctUpdate=Output Function  fctName='getRangeOfParams'  INPUT_SIZE=1  INPUT1=uint8  INPUT2=uint8  INPUT3=--  OUTPUT_SIZE=2  OUTPUT1=real32  SampleTime=.01  InputType=[ 2 2 ]  OutputType=[ 7 ]  FctDeclaration=extern void getRangeOfParams(uint8_T u1, uint8_T u2,real32_T* y1);  FctCall=getRangeOfParams(%u1, %u2, *%y1);  OrderingInOutPopup=None  FctStart=None  FctStart_Name=Init_onlyOnce  FctStart_Declaration=inline extern void Init_onlyOnce();  FctStart_Call=Init_onlyOnce();  FctInit=None  FctInit_Name=Init_Reset  FctInit_Declaration=inline extern void Init_Reset();  FctInit_Call=Init_Reset();  PinDigitalInput=[]  PinDigitalOutput=[]  AnalogueInput=[]
  "Get Range of Values [navSupport.c]  " : dsPICdrivers/OTHERS/C Function Call  Tag=dsPIC_dsPIC_CFunctionCall  FctUpdate=Output Function  fctName='getRangeOfParams'  INPUT_SIZE=1  INPUT1=uint8  INPUT2=uint8  INPUT3=--  OUTPUT_SIZE=3  OUTPUT1=real32  SampleTime=.01  InputType=[ 2 2 ]  OutputType=[ 7 ]  FctDeclaration=extern void getRangeOfParams(uint8_T u1, uint8_T u2,real32_T* y1);  FctCall=getRangeOfParams(%u1, %u2, *%y1);  OrderingInOutPopup=None  FctStart=None  FctStart_Name=Init_onlyOnce  FctStart_Declaration=inline extern void Init_onlyOnce();  FctStart_Call=Init_onlyOnce();  FctInit=None  FctInit_Name=Init_Reset  FctInit_Declaration=inline extern void Init_Reset();  FctInit_Call=Init_Reset();  PinDigitalInput=[]  PinDigitalOutput=[]  AnalogueInput=[]
  "Get Range of Values [navSupport.c]   " : dsPICdrivers/OTHERS/C Function Call  Tag=dsPIC_dsPIC_CFunctionCall  FctUpdate=Output Function  fctName='getRangeOfParams'  INPUT_SIZE=1  INPUT1=uint8  INPUT2=uint8  INPUT3=--  OUTPUT_SIZE=3  OUTPUT1=real32  SampleTime=.01  InputType=[ 2 2 ]  OutputType=[ 7 ]  FctDeclaration=extern void getRangeOfParams(uint8_T u1, uint8_T u2,real32_T* y1);  FctCall=getRangeOfParams(%u1, %u2, *%y1);  OrderingInOutPopup=None  FctStart=None  FctStart_Name=Init_onlyOnce  FctStart_Declaration=inline extern void Init_onlyOnce();  FctStart_Call=Init_onlyOnce();  FctInit=None  FctInit_Name=Init_Reset  FctInit_Declaration=inline extern void Init_Reset();  FctInit_Call=Init_Reset();  PinDigitalInput=[]  PinDigitalOutput=[]  AnalogueInput=[]
  "Get Range of Values [navSupport.c]     " : dsPICdrivers/OTHERS/C Function Call  Tag=dsPIC_dsPIC_CFunctionCall  FctUpdate=Output Function  fctName='getRangeOfParams'  INPUT_SIZE=1  INPUT1=uint8  INPUT2=uint8  INPUT3=--  OUTPUT_SIZE=3  OUTPUT1=real32  SampleTime=.01  InputType=[ 2 2 ]  OutputType=[ 7 ]  FctDeclaration=extern void getRangeOfParams(uint8_T u1, uint8_T u2,real32_T* y1);  FctCall=getRangeOfParams(%u1, %u2, *%y1);  OrderingInOutPopup=None  FctStart=None  FctStart_Name=Init_onlyOnce  FctStart_Declaration=inline extern void Init_onlyOnce();  FctStart_Call=Init_onlyOnce();  FctInit=None  FctInit_Name=Init_Reset  FctInit_Declaration=inline extern void Init_Reset();  FctInit_Call=Init_Reset();  PinDigitalInput=[]  PinDigitalOutput=[]  AnalogueInput=[]
  Get a single Param [navSupport.c] : dsPICdrivers/OTHERS/C Function Call  Tag=dsPIC_dsPIC_CFunctionCall  FctUpdate=Output Function  fctName='getParamIdx'  INPUT_SIZE=1  INPUT1=uint8  INPUT2=--  INPUT3=--  OUTPUT_SIZE=1  OUTPUT1=real32  SampleTime=.01  InputType=[ 2 ]  OutputType=[ 7 ]  FctDeclaration=extern real32_T getParamIdx(uint8_T u1);  FctCall=%y1 = getParamIdx(%u1);  OrderingInOutPopup=None  FctStart=None  FctStart_Name=Init_onlyOnce  FctStart_Declaration=inline extern void Init_onlyOnce();  FctStart_Call=Init_onlyOnce();  FctInit=None  FctInit_Name=Init_Reset  FctInit_Declaration=inline extern void Init_Reset();  FctInit_Call=Init_Reset();  PinDigitalInput=[]  PinDigitalOutput=[]  AnalogueInput=[]
  Get a single Param [navSupport.c]1 : dsPICdrivers/OTHERS/C Function Call  Tag=dsPIC_dsPIC_CFunctionCall  FctUpdate=Output Function  fctName='getParamIdx'  INPUT_SIZE=1  INPUT1=uint8  INPUT2=--  INPUT3=--  OUTPUT_SIZE=1  OUTPUT1=real32  SampleTime=.01  InputType=[ 2 ]  OutputType=[ 7 ]  FctDeclaration=extern real32_T getParamIdx(uint8_T u1);  FctCall=%y1 = getParamIdx(%u1);  OrderingInOutPopup=None  FctStart=None  FctStart_Name=Init_onlyOnce  FctStart_Declaration=inline extern void Init_onlyOnce();  FctStart_Call=Init_onlyOnce();  FctInit=None  FctInit_Name=Init_Reset  FctInit_Declaration=inline extern void Init_Reset();  FctInit_Call=Init_Reset();  PinDigitalInput=[]  PinDigitalOutput=[]  AnalogueInput=[]
  uHold PID : Outport
  he2Th PID : Outport  Port=2
  Roll2H FF : Outport  Port=3
  th2dE PID : Outport  Port=4
  Yaw Damp PID : Outport  Port=5
  Roll PID : Outport  Port=6
  dT FF : Outport  Port=7
  wires:
  Constant1/1 -> Get Range of Values [navSupport.c]/1
  Constant7/1 -> Get Range of Values [navSupport.c]/2
  Get Range of Values [navSupport.c]/1 -> uHold PID/1
  Constant6/1 -> "Get Range of Values [navSupport.c] "/1
  Constant8/1 -> "Get Range of Values [navSupport.c] "/2
  "Get Range of Values [navSupport.c] "/1 -> he2Th PID/1
  Constant9/1 -> Get a single Param [navSupport.c]/1
  Get a single Param [navSupport.c]/1 -> Roll2H FF/1
  Constant2/1 -> "Get Range of Values [navSupport.c]     "/1
  Constant3/1 -> "Get Range of Values [navSupport.c]     "/2
  "Get Range of Values [navSupport.c]     "/1 -> Roll PID/1
  Constant4/1 -> "Get Range of Values [navSupport.c]  "/1
  Constant5/1 -> "Get Range of Values [navSupport.c]  "/2
  "Get Range of Values [navSupport.c]  "/1 -> Yaw Damp PID/1
  Constant10/1 -> "Get Range of Values [navSupport.c]   "/1
  Constant11/1 -> "Get Range of Values [navSupport.c]   "/2
  "Get Range of Values [navSupport.c]   "/1 -> th2dE PID/1
  Constant12/1 -> Get a single Param [navSupport.c]1/1
  Get a single Param [navSupport.c]1/1 -> dT FF/1

== system intgratedMCUSlugs/Pilot LED and HIL Control Pins ==
  In1 : Inport
  HIL_Status : Inport  Port=2
  Data Type Conversion1 : DataTypeConversion  OutDataTypeStr=boolean
  Data Type Conversion2 : DataTypeConversion  OutDataTypeStr=boolean
  HIL Attitude  On/Off Switch : dsPICdrivers/Digital I//O/Digital Output Write  Tag=dsPIC_Digital_Output  Priority=5  PORT=B  Pin=[6]  Simultaneous=off  OrderingInOutPopup=None
  HIL On/Off Switch : dsPICdrivers/Digital I//O/Digital Output Write  Tag=dsPIC_Digital_Output  Priority=5  PORT=E  Pin=[9]  Simultaneous=off  OrderingInOutPopup=None
  Off : Constant  Value=0  OutDataTypeStr=boolean
  Terminator : Terminator
  VI Sensor DO1 : dsPICdrivers/Digital I//O/Digital Output Write  Tag=dsPIC_Digital_Output  Priority=5  PORT=G  Pin=[8]  Simultaneous=off  OrderingInOutPopup=None
  VI Sensor DO2 : dsPICdrivers/Digital I//O/Digital Output Write  Tag=dsPIC_Digital_Output  Priority=5  PORT=G  Pin=[9]  Simultaneous=off  OrderingInOutPopup=None
  wires:
  HIL_Status/1 -> Data Type Conversion1/1
  Data Type Conversion1/1 -> HIL On/Off Switch/1, HIL Attitude  On/Off Switch/1
  In1/1 -> Data Type Conversion2/1
  Data Type Conversion2/1 -> Terminator/1
  Off/1 -> VI Sensor DO1/1, VI Sensor DO2/1

== system intgratedMCUSlugs/Position and Attitude Filter ==
  A_sens(m/s^2) : Inport
  Omega (rad/s) : Inport  Port=2
  GPSMain : Inport  Port=3
  Baro Alt (m) : Inport  Port=4
  "A_sens(m/s^2) " : InportShadow  Port=1
  Attitude Complimentary Filter COG : Subsystem
  COG.SOG2V : Subsystem
  Checks if FixType is 3 [updateSensorMCUState.c] : dsPICdrivers/OTHERS/C Function Call  Tag=dsPIC_dsPIC_CFunctionCall  FctUpdate=Output Function  fctName='isFixValid'  INPUT_SIZE=1  INPUT1=--  INPUT2=--  INPUT3=--  OUTPUT_SIZE=1  OUTPUT1=uint8  SampleTime=0.01  InputType=[ ]  OutputType=[ 2 ]  FctDeclaration=extern uint8_T isFixValid();  FctCall=%y1 = isFixValid();  OrderingInOutPopup=None  FctStart=None  FctStart_Name=Init_onlyOnce  FctStart_Declaration=inline extern void Init_onlyOnce();  FctStart_Call=Init_onlyOnce();  FctInit=None  FctInit_Name=Init_Reset  FctInit_Declaration=inline extern void Init_Reset();  FctInit_Call=Init_Reset();  PinDigitalInput=[]  PinDigitalOutput=[]  AnalogueInput=[]
  Compute GS Location : Subsystem
  Demux : Demux  Outputs=5
  Enabled Subsystem : Subsystem  TreatAsAtomicUnit=on
  GPS Update : Subsystem  mask{T=0.01}
      mask prompts: T "Sample Time"
  Geod2LTP1 : Subsystem
      mask Description:
      | This block provides transformation of the Geodetic coordinates
      | to the LTP coorinate system. The block uses two consecutive transformations
      | (Geodetic -> ECEF ->LTP).
      | Geodetic coordinates of the LTP origin should also be predetermined.
      mask Help: Oops!
      mask Display: plot(0,0,100,100,[45,40,35,40,40],[85,95,85,95,40],[85,95,85,95,40],[35,40,45,40,40],[60,40,10,20,10,14],[70,40,10,13,10,20],[56,45],[70,70],[60,60],[50,60],[60,60],[30,40],[50,60],[20,20],[30,40],[20,20],[45,55],[35,25],[75,65],[35,25])
  Get the GS Location [updateSensorMCUState.c] : dsPICdrivers/OTHERS/C Function Call  Tag=dsPIC_dsPIC_CFunctionCall  FctUpdate=Output Function  fctName='getGSLocation'  INPUT_SIZE=1  INPUT1=--  INPUT2=--  INPUT3=--  OUTPUT_SIZE=3  OUTPUT1=real32  SampleTime=0.01  InputType=[ ]  OutputType=[ 7 ]  FctDeclaration=extern void getGSLocation(real32_T* y1);  FctCall=getGSLocation(*%y1);  OrderingInOutPopup=None  FctStart=None  FctStart_Name=Init_onlyOnce  FctStart_Declaration=inline extern void Init_onlyOnce();  FctStart_Call=Init_onlyOnce();  FctInit=None  FctInit_Name=Init_Reset  FctInit_Declaration=inline extern void Init_Reset();  FctInit_Call=Init_Reset();  PinDigitalInput=[]  PinDigitalOutput=[]  AnalogueInput=[]
  Position Filter : Subsystem
  "[1 1 -1]" : Gain  Gain=[1 1 -1]
  get Height : Selector  InputPortWidth=3  IndexOptions=Index vector (dialog)  Indices=[1]  OutputSizes=1
  euler_hat (rad) : Outport
  pqr_hat (rad/s) : Outport  Port=2
  Pxyz_hat (m) : Outport  Port=3
  Vned_hat (m/s) : Outport  Port=4
  GyroBias (rad/s) : Outport  Port=5
  Accel Bias (m/s) : Outport  Port=6
  wires:
  Position Filter/1(Vxyd_hat) -> Vned_hat (m/s)/1, Attitude Complimentary Filter COG/4(Vxyd_hat)
  Position Filter/2(Pxyd_hat) -> Pxyz_hat (m)/1
  Position Filter/3(acc_bias) -> Accel Bias (m/s)/1, Attitude Complimentary Filter COG/5(acc_bias)
  Attitude Complimentary Filter COG/1(euler_hat) -> euler_hat (rad)/1
  Attitude Complimentary Filter COG/2(pqr_hat) -> pqr_hat (rad/s)/1
  Attitude Complimentary Filter COG/3(Gyro Bias) -> GyroBias (rad/s)/1
  GPSMain/1 -> Demux/1
  Get the GS Location [updateSensorMCUState.c]/1 -> Compute GS Location/1(GS Location), get Height/1
  Demux/1 -> Geod2LTP1/3("Lat, deg(GPS)")
  Demux/2 -> Geod2LTP1/4("Lon, deg(GPS)")
  Demux/3 -> Geod2LTP1/5(Hight,m(GPS))
  Compute GS Location/2(R_in) -> Geod2LTP1/2(GS ECEF)
  Compute GS Location/1("Lat, Lon") -> Geod2LTP1/1(GS Lat,Lon)
  GPS Update/1(Update?) -> Position Filter/1(NewGPS)
  A_sens(m/s^2)/1 -> Attitude Complimentary Filter COG/1(A_sens)
  Omega (rad/s)/1 -> Attitude Complimentary Filter COG/3(Gyros)
  "[1 1 -1]"/1 -> Position Filter/4(GPS_XYD)
  [XY_Orient] -> Attitude Complimentary Filter COG/2(XY Orient)
  Baro Alt (m)/1 -> Position Filter/2(Baro Alt)
  COG.SOG2V/1(Vnorth) -> Position Filter/5(Vnorth)
  COG.SOG2V/2(Veast) -> Position Filter/6(Veast)
  COG.SOG2V/3(XY Orient) -> [XY_Orient]
  Checks if FixType is 3 [updateSensorMCUState.c]/1 -> Enabled Subsystem/Enable
  Attitude Complimentary Filter COG/4(RL2B) -> [RL2B]
  [RL2B] -> Position Filter/3(RLT2B)
  Enabled Subsystem/1(Out1) -> GPS Update/1(XYZ), "[1 1 -1]"/1
  Geod2LTP1/1("NEU, m") -> Enabled Subsystem/1(In1)
  Demux/4 -> Enabled Subsystem/2(In2)
  Demux/5 -> Enabled Subsystem/3(In3)
  Enabled Subsystem/2(Out2) -> COG.SOG2V/1(COG_D)
  Enabled Subsystem/3(Out3) -> COG.SOG2V/2(SOG), Position Filter/7(SOG)
  "A_sens(m/s^2) "/1 -> Position Filter/8(A_sens(m/s^2))
  get Height/1 -> Position Filter/9(Base Height (m))

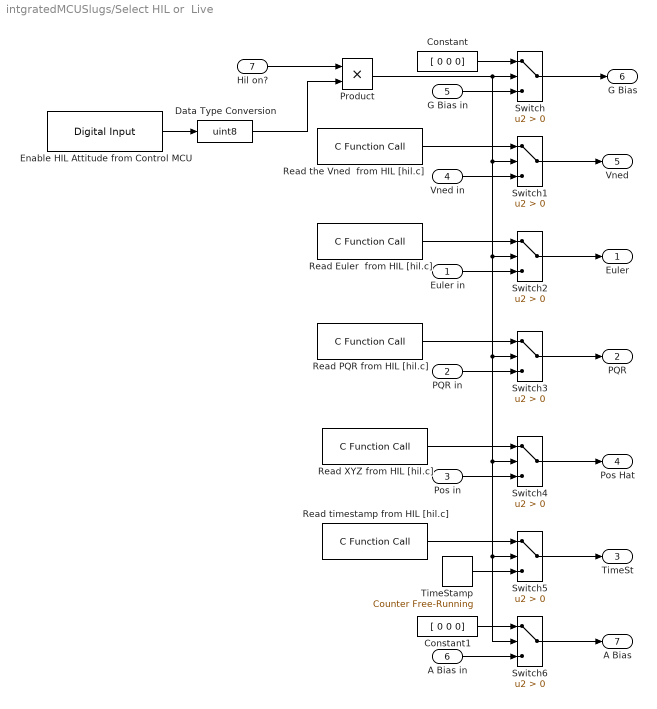
== system intgratedMCUSlugs/Select HIL or  Live ==
  Euler in : Inport
  PQR in : Inport  Port=2
  Pos in : Inport  Port=3
  Vned in : Inport  Port=4
  G Bias in : Inport  Port=5
  A Bias in : Inport  Port=6
  Hil on? : Inport  Port=7
  Constant : Constant  Value=[ 0 0 0]  OutDataTypeStr=single
  Constant1 : Constant  Value=[ 0 0 0]  OutDataTypeStr=single
  Data Type Conversion : DataTypeConversion  OutDataTypeStr=uint8
  Enable HIL Attitude from Control MCU : dsPICdrivers/Digital I//O/Digital Input  Tag=dsPIC_Digital_Input  PORT=A  Pin=[14]  SampleTime=.01  OrderingInOutPopup=None
  Product : Product  OutDataTypeStr=uint8  RndMeth=Zero
  Read Euler  from HIL [hil.c] : dsPICdrivers/OTHERS/C Function Call  Tag=dsPIC_dsPIC_CFunctionCall  FctUpdate=Output Function  fctName='hil_getEuler'  INPUT_SIZE=1  INPUT1=--  INPUT2=--  INPUT3=--  OUTPUT_SIZE=3  OUTPUT1=real32  SampleTime=.01  InputType=[ ]  OutputType=[ 7 ]  FctDeclaration=extern void hil_getEuler(real32_T* y1);  FctCall=hil_getEuler(*%y1);  OrderingInOutPopup=None  FctStart=None  FctStart_Name=Init_onlyOnce  FctStart_Declaration=inline extern void Init_onlyOnce();  FctStart_Call=Init_onlyOnce();  FctInit=None  FctInit_Name=Init_Reset  FctInit_Declaration=inline extern void Init_Reset();  FctInit_Call=Init_Reset();  PinDigitalInput=[]  PinDigitalOutput=[]  AnalogueInput=[]
  Read PQR from HIL [hil.c] : dsPICdrivers/OTHERS/C Function Call  Tag=dsPIC_dsPIC_CFunctionCall  FctUpdate=Output Function  fctName='hil_getRates'  INPUT_SIZE=1  INPUT1=--  INPUT2=--  INPUT3=--  OUTPUT_SIZE=3  OUTPUT1=real32  SampleTime=.01  InputType=[ ]  OutputType=[ 7 ]  FctDeclaration=extern void hil_getRates(real32_T* y1);  FctCall=hil_getRates(*%y1);  OrderingInOutPopup=None  FctStart=None  FctStart_Name=Init_onlyOnce  FctStart_Declaration=inline extern void Init_onlyOnce();  FctStart_Call=Init_onlyOnce();  FctInit=None  FctInit_Name=Init_Reset  FctInit_Declaration=inline extern void Init_Reset();  FctInit_Call=Init_Reset();  PinDigitalInput=[]  PinDigitalOutput=[]  AnalogueInput=[]
  Read XYZ from HIL [hil.c] : dsPICdrivers/OTHERS/C Function Call  Tag=dsPIC_dsPIC_CFunctionCall  FctUpdate=Output Function  fctName='hil_getXYZ'  INPUT_SIZE=1  INPUT1=--  INPUT2=--  INPUT3=--  OUTPUT_SIZE=3  OUTPUT1=real32  SampleTime=.01  InputType=[ ]  OutputType=[ 7 ]  FctDeclaration=extern void hil_getXYZ(real32_T* y1);  FctCall=hil_getXYZ(*%y1);  OrderingInOutPopup=None  FctStart=None  FctStart_Name=Init_onlyOnce  FctStart_Declaration=inline extern void Init_onlyOnce();  FctStart_Call=Init_onlyOnce();  FctInit=None  FctInit_Name=Init_Reset  FctInit_Declaration=inline extern void Init_Reset();  FctInit_Call=Init_Reset();  PinDigitalInput=[]  PinDigitalOutput=[]  AnalogueInput=[]
  Read the Vned  from HIL [hil.c] : dsPICdrivers/OTHERS/C Function Call  Tag=dsPIC_dsPIC_CFunctionCall  FctUpdate=Output Function  fctName='hil_getVned'  INPUT_SIZE=1  INPUT1=--  INPUT2=--  INPUT3=--  OUTPUT_SIZE=3  OUTPUT1=real32  SampleTime=.01  InputType=[ ]  OutputType=[ 7 ]  FctDeclaration=extern void hil_getVned(real32_T* y1);  FctCall=hil_getVned(*%y1);  OrderingInOutPopup=None  FctStart=None  FctStart_Name=Init_onlyOnce  FctStart_Declaration=inline extern void Init_onlyOnce();  FctStart_Call=Init_onlyOnce();  FctInit=None  FctInit_Name=Init_Reset  FctInit_Declaration=inline extern void Init_Reset();  FctInit_Call=Init_Reset();  PinDigitalInput=[]  PinDigitalOutput=[]  AnalogueInput=[]
  Read timestamp from HIL [hil.c] : dsPICdrivers/OTHERS/C Function Call  Tag=dsPIC_dsPIC_CFunctionCall  FctUpdate=Output Function  fctName='hil_getTs'  INPUT_SIZE=1  INPUT1=--  INPUT2=--  INPUT3=--  OUTPUT_SIZE=1  OUTPUT1=int32  SampleTime=.01  InputType=[ ]  OutputType=[ 5 ]  FctDeclaration=extern int32_T hil_getTs();  FctCall=%y1 = hil_getTs();  OrderingInOutPopup=None  FctStart=None  FctStart_Name=Init_onlyOnce  FctStart_Declaration=inline extern void Init_onlyOnce();  FctStart_Call=Init_onlyOnce();  FctInit=None  FctInit_Name=Init_Reset  FctInit_Declaration=inline extern void Init_Reset();  FctInit_Call=Init_Reset();  PinDigitalInput=[]  PinDigitalOutput=[]  AnalogueInput=[]
  Switch{,1..6} (7 alike) : Switch  Criteria=u2 > Threshold
  TimeStamp : simulink/Sources/Counter Free-Running  NumBits=32  tsamp=.01
  Euler : Outport
  PQR : Outport  Port=2
  TimeSt : Outport  Port=3
  Pos Hat : Outport  Port=4
  Vned : Outport  Port=5
  G Bias : Outport  Port=6
  A Bias : Outport  Port=7
  wires:
  Switch/1 -> G Bias/1
  Constant/1 -> Switch/1
  Product/1 -> Switch/2, Switch1/2, Switch2/2, Switch3/2, Switch4/2, Switch5/2, Switch6/2
  G Bias in/1 -> Switch/3
  Switch1/1 -> Vned/1
  Read the Vned  from HIL [hil.c]/1 -> Switch1/1
  Vned in/1 -> Switch1/3
  Read Euler  from HIL [hil.c]/1 -> Switch2/1
  Euler in/1 -> Switch2/3
  Switch2/1 -> Euler/1
  Read PQR from HIL [hil.c]/1 -> Switch3/1
  PQR in/1 -> Switch3/3
  Switch3/1 -> PQR/1
  Read XYZ from HIL [hil.c]/1 -> Switch4/1
  Pos in/1 -> Switch4/3
  Switch4/1 -> Pos Hat/1
  TimeStamp/1 -> Switch5/3
  Read timestamp from HIL [hil.c]/1 -> Switch5/1
  Enable HIL Attitude from Control MCU/1 -> Data Type Conversion/1
  Hil on?/1 -> Product/1
  Data Type Conversion/1 -> Product/2
  Switch5/1 -> TimeSt/1
  Switch6/1 -> A Bias/1
  Constant1/1 -> Switch6/1
  A Bias in/1 -> Switch6/3

== system intgratedMCUSlugs/Sensor Data ==
  Data Type Conversion : DataTypeConversion  OutDataTypeStr=uint8  SampleTime=0.01
  Enable HIL from  Control MCU : dsPICdrivers/Digital I//O/Digital Input  Tag=dsPIC_Digital_Input  PORT=D  Pin=[2]  SampleTime=.01  OrderingInOutPopup=None
  Raw HIL  Readings : Subsystem
  Sensor Suite : Subsystem
  Omega (rad/s) : Outport
  Accel (m/s^2) : Outport  Port=2
  Mag (mG) : Outport  Port=3
  Baro Alt (m) : Outport  Port=4
  HIL On? : Outport  Port=5
  GPS : Outport  Port=6
  wires:
  Raw HIL  Readings/1(Raw Msg) -> Sensor Suite/2(Raw HIL)
  Enable HIL from  Control MCU/1 -> Raw HIL  Readings/Enable, Sensor Suite/1(D2), Data Type Conversion/1
  Data Type Conversion/1 -> HIL On?/1
  Sensor Suite/1(Omega (rad/s)) -> Omega (rad/s)/1
  Sensor Suite/2(Accel (m/s^2)) -> Accel (m/s^2)/1
  Sensor Suite/3(Mag (mG)) -> Mag (mG)/1
  Sensor Suite/4(Baro Alt (m)) -> Baro Alt (m)/1
  Sensor Suite/5(GPS) -> GPS/1
